simulink model "PR_TestDemo"  (R2017a)
settings: Solver=VariableStepAuto  StartTime=0.0  StopTime=1  RelTol=1e-3
InitFcn:
  | Ts_Control = 1e-4;
  | Kp = 0 ;
  | Kr = 10 ;
  | wi = pi ;
undefined symbols (not defined in the file or in its folder): DiscIntNeverNeededParam
settings Model: Creator=donghao  LastModifiedBy=donghao

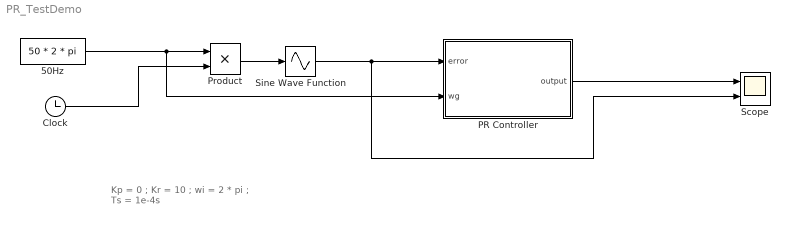
== system PR_TestDemo ==
  note: Kp = 0 ;
      | Kr = 10 ;
      | wi = 2 * pi ;
      | Ts = 1e-4s
  50Hz : Constant  Value=50 * 2 * pi
  Clock : Clock
  PR Controller : Subsystem
  Product : Product
  Scope : Scope  NumInputPorts=2
  Sine Wave Function : Sin  TimeSource=Use external signal  SampleTime=0
  wires:
  Product/1 -> Sine Wave Function/1
  50Hz/1 -> PR Controller/2(wg), Product/1
  Clock/1 -> Product/2
  Sine Wave Function/1 -> PR Controller/1(error), Scope/2
  PR Controller/1(output) -> Scope/1

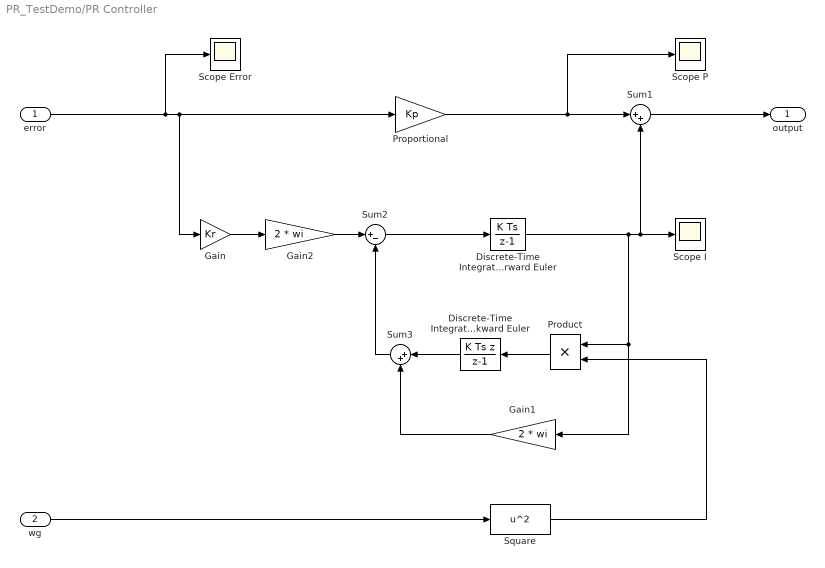
== system PR_TestDemo/PR Controller ==
  error : Inport
  wg : Inport  Port=2
  Discrete-Time Integrator-Backward Euler : DiscreteIntegrator  IntegratorMethod=Integration: Backward Euler  InitialConditionSetting=State (most efficient)  SampleTime=Ts_Control  ICPrevOutput=DiscIntNeverNeededParam  ICPrevScaledInput=DiscIntNeverNeededParam
  Discrete-Time Integrator-Forward Euler : DiscreteIntegrator  InitialConditionSetting=State (most efficient)  SampleTime=Ts_Control  ICPrevOutput=DiscIntNeverNeededParam  ICPrevScaledInput=DiscIntNeverNeededParam
  Gain : Gain  Gain=Kr
  Gain1 : Gain  Gain=2 * wi
  Gain2 : Gain  Gain=2 * wi
  Product : Product
  Proportional : Gain  Gain=Kp
  Scope Error : Scope
  Scope I : Scope
  Scope P : Scope
  Square : Fcn  Expr=u^2
  Sum1 : Sum  Inputs=|++
  Sum2 : Sum  Inputs=|+-
  Sum3 : Sum  Inputs=|++
  output : Outport
  wires:
  Discrete-Time Integrator-Forward Euler/1 -> Gain1/1, Product/1, Sum1/2, Scope I/1
  Sum1/1 -> output/1
  error/1 -> Scope Error/1, Proportional/1, Gain/1
  Proportional/1 -> Scope P/1, Sum1/1
  Gain/1 -> Gain2/1
  Sum2/1 -> Discrete-Time Integrator-Forward Euler/1
  Product/1 -> Discrete-Time Integrator-Backward Euler/1
  wg/1 -> Square/1
  Square/1 -> Product/2
  Discrete-Time Integrator-Backward Euler/1 -> Sum3/1
  Gain1/1 -> Sum3/2
  Gain2/1 -> Sum2/1
  Sum3/1 -> Sum2/2
